simulink model "oven_test_LCO_0D_2020a"  (R2020a)
settings: Solver=VariableStepAuto  StartTime=0.0  StopTime=3600  RelTol=1e-6
settings Model: Creator=jostanek  LastModifiedBy=jostanek

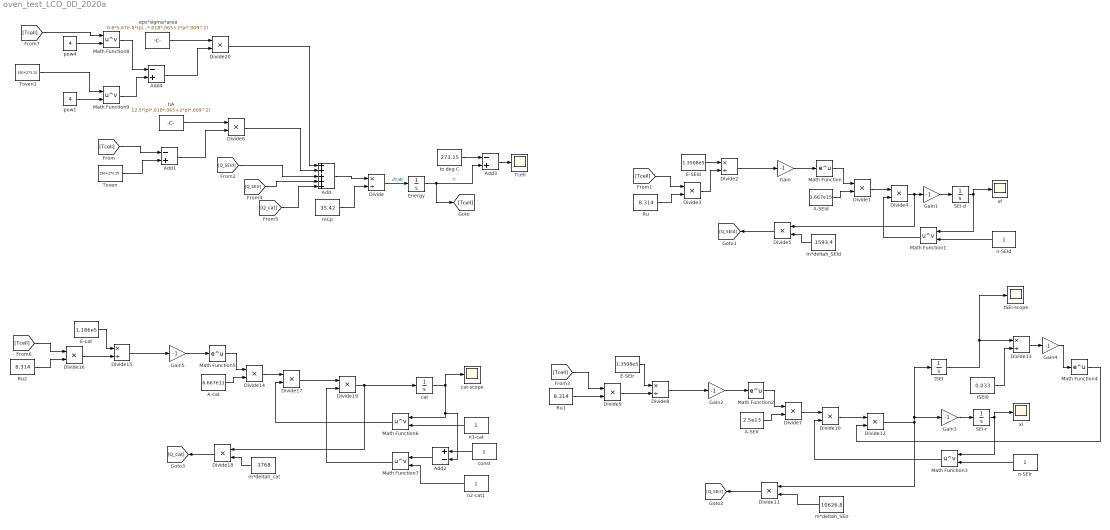
== system oven_test_LCO_0D_2020a ==
  A-SEId : Constant  Value=1.667e15
  A-SEIr : Constant  Value=2.5e13
  A-cat : Constant  Value=6.667e11
  Add : Sum  Inputs=+++++
  Add1 : Sum  Inputs=-+
  Add2 : Sum  Inputs=+-
  Add3 : Sum  Inputs=-+
  Add4 : Sum  Inputs=-+
  Divide{,2,8,13,15} (5 alike) : Product  Inputs=*/
  Divide{1,3..7,9..12,14,16..20} (16 alike) : Product  Inputs=**
  E-SEId : Constant  Value=1.3508e5
  E-SEIr : Constant  Value=1.3508e5
  E-cat : Constant  Value=1.186e5
  Energy : Integrator  InitialCondition=293.15
  Gain{,1..5} (6 alike) : Gain  Gain=-1
  Math Function{,2,4..5} (4 alike) : Math  SaturateOnIntegerOverflow=on
  Math Function{1,3,6..9} (6 alike) : Math  Operator=pow  SaturateOnIntegerOverflow=on
  Ru : Constant  Value=8.314
  Ru1 : Constant  Value=8.314
  Ru2 : Constant  Value=8.314
  SEI-d : Integrator  InitialCondition=0.15
  SEI-r : Integrator  InitialCondition=.75
  Tcell : Scope
  Toven : Constant  Value=150+273.15
  Toven1 : Constant  Value=150+273.15
  cat : Integrator  InitialCondition=.04
  cat-scope : Scope
  const : Constant
  eps*sigma*area : Constant  Value=0.8*5.67e-8*(pi*.018*.065+2*pi*.009^2)
  hA : Constant  Value=12.5*(pi*.018*.065+2*pi*.009^2)
  m*deltah_SEId : Constant  Value=1593.4
  m*deltah_SEIr : Constant  Value=10626.8
  m*deltah_cat : Constant  Value=3768
  mCp : Constant  Value=35.42
  n-SEId : Constant
  n-SEIr : Constant
  n1-cat : Constant
  n2-cat1 : Constant
  pow1 : Constant  Value=4
  pow4 : Constant  Value=4
  tSEI : Integrator  InitialCondition=0.033
  tSEI-scope : Scope
  tSEI0 : Constant  Value=0.033
  to deg C : Constant  Value=273.15
  xf : Scope
  xi : Scope
  wires:
  mCp/1 -> Divide/2
  Divide/1 -> Energy/1  "dT/dt"
  Math Function/1 -> Divide1/1
  A-SEId/1 -> Divide1/2
  E-SEId/1 -> Divide2/1
  Ru/1 -> Divide3/2
  Divide3/1 -> Divide2/2
  Divide2/1 -> Gain/1
  Gain/1 -> Math Function/1
  SEI-d/1 -> xf/1, Math Function1/1
  n-SEId/1 -> Math Function1/2
  Math Function1/1 -> Divide4/2
  m*deltah_SEId/1 -> Divide5/2
  hA/1 -> Divide6/1
  Add/1 -> Divide/1
  Divide4/1 -> Divide5/1, Gain1/1
  Divide1/1 -> Divide4/1
  Gain1/1 -> SEI-d/1
  Toven/1 -> Add1/2
  Add1/1 -> Divide6/2
  Divide6/1 -> Add/2
  Gain3/1 -> SEI-r/1
  Divide7/1 -> Divide10/1
  Math Function3/1 -> Divide10/2
  n-SEIr/1 -> Math Function3/2
  SEI-r/1 -> Math Function3/1, xi/1
  Gain2/1 -> Math Function2/1
  Divide8/1 -> Gain2/1
  Divide9/1 -> Divide8/2
  Ru1/1 -> Divide9/2
  E-SEIr/1 -> Divide8/1
  A-SEIr/1 -> Divide7/2
  Math Function2/1 -> Divide7/1
  m*deltah_SEIr/1 -> Divide11/2
  Divide10/1 -> Divide12/1
  Divide12/1 -> tSEI/1, Gain3/1, Divide11/1
  tSEI/1 -> tSEI-scope/1, Divide13/1
  tSEI0/1 -> Divide13/2
  Divide13/1 -> Gain4/1
  Gain4/1 -> Math Function4/1
  Math Function4/1 -> Divide12/2
  Energy/1 -> Add3/2, [Tcell]  "T"
  Divide19/1 -> cat/1, Divide18/1
  Divide14/1 -> Divide17/1
  m*deltah_cat/1 -> Divide18/2
  Math Function6/1 -> Divide17/2
  n1-cat/1 -> Math Function6/2
  cat/1 -> cat-scope/1, Add2/2, Math Function6/1
  Gain5/1 -> Math Function5/1
  Divide15/1 -> Gain5/1
  Divide16/1 -> Divide15/2
  Ru2/1 -> Divide16/2
  E-cat/1 -> Divide15/1
  A-cat/1 -> Divide14/2
  Math Function5/1 -> Divide14/1
  Divide17/1 -> Divide19/1
  const/1 -> Add2/1
  n2-cat1/1 -> Math Function7/2
  Add2/1 -> Math Function7/1
  Math Function7/1 -> Divide19/2
  [Tcell] -> Add1/1
  [Tcell] -> Divide3/1
  Divide5/1 -> [Q_SEId]
  [Q_SEId] -> Add/3
  [Tcell] -> Divide9/1
  Divide11/1 -> [Q_SEIr]
  [Q_SEIr] -> Add/4
  Divide18/1 -> [Q_cat]
  [Tcell] -> Divide16/1
  to deg C/1 -> Add3/1
  Add3/1 -> Tcell/1
  Add4/1 -> Divide20/2
  eps*sigma*area/1 -> Divide20/1
  Divide20/1 -> Add/1
  pow4/1 -> Math Function8/2
  [Tcell] -> Math Function8/1
  Math Function8/1 -> Add4/1
  Toven1/1 -> Math Function9/1
  pow1/1 -> Math Function9/2
  Math Function9/1 -> Add4/2
  [Q_cat] -> Add/5
